simulink model "Week3Challengeq2_1640261440"  (R2021b)
settings: Solver=VariableStepAuto  StartTime=0.0  StopTime=10.0  RelTol=1e-3
values from neighbouring files (symbols this model uses):
  x = [22 3 55.6 9 12 10]    [week3Challenge2_1640261395.mat]
  y = [5 31 95 56.3 77 61]    [week3Challenge2_1640261395.mat]
settings Model: Creator=Ish  LastModifiedBy=Ish
settings DataIOCC: ExternalInput=[x, y]

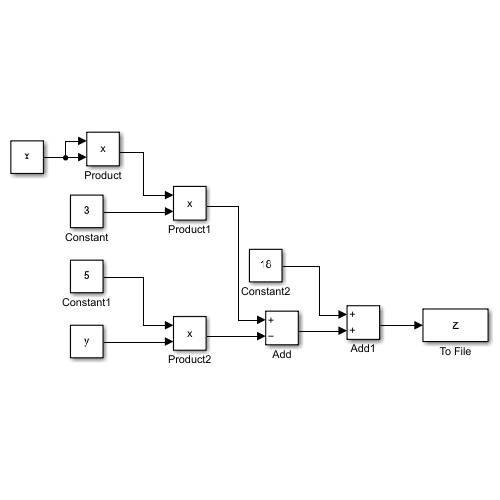
[thumbnail: Simulink's stored preview of the top-level diagram]
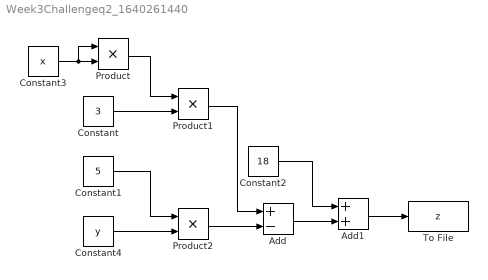
== system Week3Challengeq2_1640261440 ==
  Add : Sum  Inputs=+-
  Add1 : Sum
  Constant : Constant  Value=3
  Constant1 : Constant  Value=5
  Constant2 : Constant  Value=18
  Constant3 : Constant  Value=x
  Constant4 : Constant  Value=y
  Product : Product
  Product1 : Product
  Product2 : Product
  To File : ToFile  Filename=z
  wires:
  Constant4/1 -> Product2/2
  Product2/1 -> Add/2
  Product1/1 -> Add/1
  Add1/1 -> To File/1
  Product/1 -> Product1/1
  Add/1 -> Add1/2
  Constant2/1 -> Add1/1
  Constant/1 -> Product1/2
  Constant1/1 -> Product2/1
  Constant3/1 -> Product/2, Product/1
